simulink model "Motion_planner_Street_Drone"  (R2019b)
settings: Solver=FixedStepAuto  StartTime=0.0  StopTime=25  FixedStep=0.0075  MaxStep=1e-1  MinStep=1e-3  RelTol=1e-3  AbsTol=1e-4
InitFcn:
  | SD_init1
values from neighbouring files (symbols this model uses):
  cost = [2.71432892747 3.32441927977 3.79268757264 4.85642115368 6.12135035287 7.09825974303 9.57278659789 1.55754789407 1.51399555616 2.57723707661 3.8468529147 4.8336387623 ... (2430 elements, 1x2430)]    [matlab.mat]
  Front_brake = [0 2.2085352751 4.15209150797 6.12733711785 8.16604105928 9.79119154879 12.1808659635 14.1242630413 16.1155522836 18.1386900579 20.0839213981 22.1313006548 ... (68 elements, 34x2)]    [Front_brake.mat]
  N = size(X,1)    [curvature.m]
  obsx = [dx1 dx2 dx3 dx4]'    [dynamic_collison.m]    (also in dynamic_detection1.m = [x1 x2 x3 x4]')
  obsy = [dy1 dy2 dy3 dy4]'    [dynamic_collison.m]    (also in dynamic_detection1.m = [y1 y2 y3 y4]')
  x = obs_path(i,1)    [dynamic_collison.m]    (also in dynamic_detection1.m)
  X = [X]    [curvature.m]
  y = obs_path(i,2)    [dynamic_collison.m]    (also in dynamic_detection1.m)
undefined symbols (not defined in the file or in its folder): d, dfin, dini, Ki, Kp, L_0f, lookahead_time, lookahead_time_rev, Rear_brake, sigbuilder_block, steer_ratio, steer_sens, tfin, tini, TPS_0, xfin, Y, yfin, Z
libraries: sm_lib x290, nesl_utility x136, simulink x6, vrlib x2, powerlib_meascontrol x2
(part 1 of 14)
settings Model: PacingRate=0.320000  Creator=dpawa  LastModifiedBy=prave
settings SolverCC: AutoScaleAbsTol=off  InitialStep=1e-2  ZeroCrossAlgorithm=Adaptive  AlgebraicLoopSolver=LineSearch
settings DebuggingCC: AlgebraicLoopMsg=none  MaskedZcDiagnostic=none  IgnoredZcDiagnostic=none  UnderSpecifiedDimensionMsg=warning

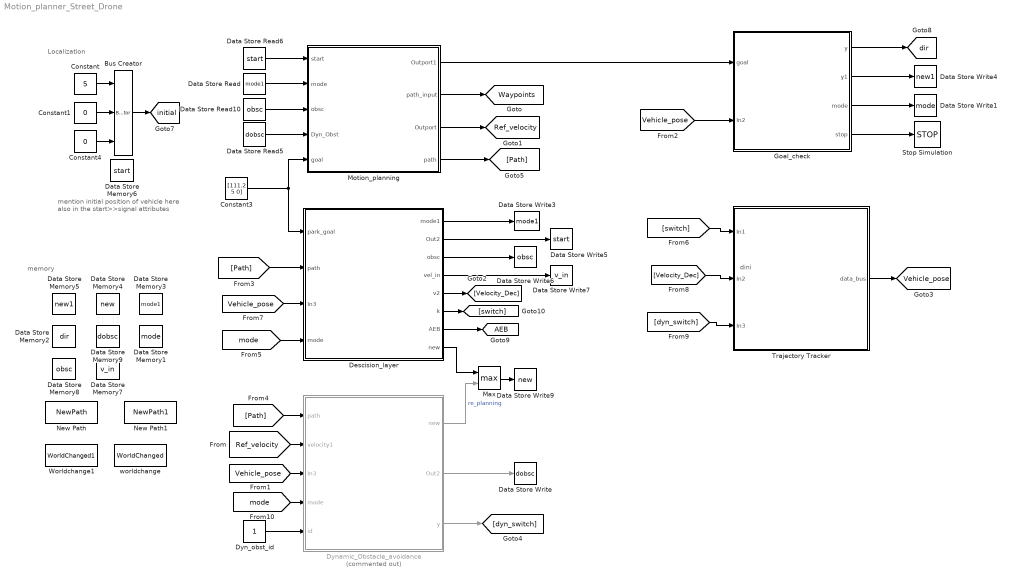
== system Motion_planner_Street_Drone ==
  note: dini
  note: mention initial position of vehicle here
      |  also in the start>>signal attributes
  note: Localization
  note: memory
  Bus Creator : BusCreator  Inputs=3
  Constant : Constant  Value=5
  Constant1 : Constant  Value=0
  Constant3 : Constant  Value=[111.2 5 0]
  Constant4 : Constant  Value=0
  Data Store Memory1 : DataStoreMemory  DataStoreName=mode  ReadBeforeWriteMsg=warning  WriteAfterWriteMsg=warning  WriteAfterReadMsg=warning  InitialValue=1  ShowAdditionalParam=off
  Data Store Memory2 : DataStoreMemory  DataStoreName=dir  ReadBeforeWriteMsg=warning  WriteAfterWriteMsg=warning  WriteAfterReadMsg=warning  InitialValue=1  ShowAdditionalParam=off
  Data Store Memory3 : DataStoreMemory  DataStoreName=mode1  ReadBeforeWriteMsg=warning  WriteAfterWriteMsg=warning  WriteAfterReadMsg=warning  InitialValue=2  ShowAdditionalParam=off  OutDataTypeStr=double
  Data Store Memory4 : DataStoreMemory  DataStoreName=new  ReadBeforeWriteMsg=warning  WriteAfterWriteMsg=warning  WriteAfterReadMsg=warning  ShowAdditionalParam=off  OutDataTypeStr=double
  Data Store Memory5 : DataStoreMemory  DataStoreName=new1  ReadBeforeWriteMsg=warning  WriteAfterWriteMsg=warning  WriteAfterReadMsg=warning  ShowAdditionalParam=off
  Data Store Memory6 : DataStoreMemory  DataStoreName=start  ReadBeforeWriteMsg=warning  WriteAfterWriteMsg=warning  WriteAfterReadMsg=warning  InitialValue=[5 0 0]  ShowAdditionalParam=off  OutDataTypeStr=double
  Data Store Memory7 : DataStoreMemory  DataStoreName=v_in  ReadBeforeWriteMsg=warning  WriteAfterWriteMsg=warning  WriteAfterReadMsg=warning  ShowAdditionalParam=off
  Data Store Memory8 : DataStoreMemory  DataStoreName=obsc  ReadBeforeWriteMsg=warning  WriteAfterWriteMsg=warning  WriteAfterReadMsg=warning  InitialValue=2  ShowAdditionalParam=off
  Data Store Memory9 : DataStoreMemory  DataStoreName=dobsc  ReadBeforeWriteMsg=warning  WriteAfterWriteMsg=warning  WriteAfterReadMsg=warning  InitialValue=[inf inf inf]  ShowAdditionalParam=off
  Data Store Read : DataStoreRead  DataStoreName=mode1
  Data Store Read10 : DataStoreRead  DataStoreName=obsc
  Data Store Read5 : DataStoreRead  DataStoreName=dobsc
  Data Store Read6 : DataStoreRead  DataStoreName=start  SampleTime=0.0075
  Data Store Write : DataStoreWrite  DataStoreName=dobsc
  Data Store Write1 : DataStoreWrite  DataStoreName=mode
  Data Store Write3 : DataStoreWrite  DataStoreName=mode1
  Data Store Write4 : DataStoreWrite  DataStoreName=new1
  Data Store Write5 : DataStoreWrite  DataStoreName=start  SampleTime=0.0075
  Data Store Write6 : DataStoreWrite  DataStoreName=obsc
  Data Store Write7 : DataStoreWrite  DataStoreName=v_in
  Data Store Write9 : DataStoreWrite  DataStoreName=new
  Descision_layer : Subsystem
  Dyn_obst_id : Constant
  Dynamic_Obstacle_avoidance : Subsystem  Commented=on
  Goal_check : Subsystem
  Max : MinMax  Function=max  Inputs=2
  Motion_planning : Subsystem
  "New Path " : DataStoreMemory  DataStoreName=NewPath  ReadBeforeWriteMsg=warning  WriteAfterWriteMsg=warning  WriteAfterReadMsg=warning  VectorParams1D=off  ShowAdditionalParam=off
  New Path1 : DataStoreMemory  DataStoreName=NewPath1  ReadBeforeWriteMsg=warning  WriteAfterWriteMsg=warning  WriteAfterReadMsg=warning  VectorParams1D=off  ShowAdditionalParam=off
  Stop Simulation : Stop
  Trajectory Tracker : Subsystem
  Worldchange1 : DataStoreMemory  DataStoreName=WorldChanged1  VectorParams1D=off  ShowAdditionalParam=off
  worldchange : DataStoreMemory  DataStoreName=WorldChanged  InitialValue=1  VectorParams1D=off  ShowAdditionalParam=off
  tag scope: AEB=global, Ref_velocity=global, Vehicle_pose=global, Waypoints=global, dir=global, initial=global
  wires:
  Constant3/1 -> Descision_layer/1(park_goal), Motion_planning/5(goal)
  Motion_planning/2(path_input) -> [Waypoints]
  Max/1 -> Data Store Write9/1
  [Vehicle_pose] -> Goal_check/2(In2)
  Goal_check/1(y) -> [dir]
  Goal_check/2(y1) -> Data Store Write4/1
  Goal_check/3(mode) -> Data Store Write1/1
  Goal_check/4(stop) -> Stop Simulation/1
  Data Store Read6/1 -> Motion_planning/1(start)
  Data Store Read/1 -> Motion_planning/2(mode)
  Data Store Read10/1 -> Motion_planning/3(obsc)
  Data Store Read5/1 -> Motion_planning/4(Dyn_Obst)
  Motion_planning/3(Outport) -> [Ref_velocity]
  Motion_planning/1(Outport1) -> Goal_check/1(goal)
  Dynamic_Obstacle_avoidance/1(new) -> Max/2  "re_planning"
  [Path] -> Dynamic_Obstacle_avoidance/1(path)
  [Ref_velocity] -> Dynamic_Obstacle_avoidance/2(velocity1)
  [Vehicle_pose] -> Dynamic_Obstacle_avoidance/3(In3)
  [mode] -> Dynamic_Obstacle_avoidance/4(mode)
  Dyn_obst_id/1 -> Dynamic_Obstacle_avoidance/5(id)
  Dynamic_Obstacle_avoidance/2(Out2) -> Data Store Write/1
  [Vehicle_pose] -> Descision_layer/3(In3)
  [mode] -> Descision_layer/4(mode)
  Descision_layer/1(mode1) -> Data Store Write3/1
  Descision_layer/2(Out2) -> Data Store Write5/1
  Descision_layer/3(obsc) -> Data Store Write6/1
  Descision_layer/4(vel_in) -> Data Store Write7/1
  Descision_layer/8(new) -> Max/1
  Constant1/1 -> Bus Creator/2
  Constant/1 -> Bus Creator/1
  Bus Creator/1 -> [initial]
  Constant4/1 -> Bus Creator/3
  Motion_planning/4(path) -> [Path]
  [Path] -> Descision_layer/2(path)
  Descision_layer/5(v2) -> [Velocity_Dec]
  Descision_layer/6(k) -> [switch]
  Dynamic_Obstacle_avoidance/3(y) -> [dyn_switch]
  Descision_layer/7(AEB) -> [AEB]
  [switch] -> Trajectory Tracker/1(In1)
  [Velocity_Dec] -> Trajectory Tracker/2(In2)
  [dyn_switch] -> Trajectory Tracker/3(In3)
  Trajectory Tracker/1(data_bus) -> [Vehicle_pose]

== system Motion_planner_Street_Drone/Descision_layer ==
  park_goal : Inport
  path : Inport  Port=2
  In3 : Inport  Port=3
  mode : Inport  Port=4
  Bus Selector1 : BusSelector  OutputSignals=pos.drive_x,pos.drive_y,angle.yawangle,vel.velocity_drive
  Mux : Mux  Inputs=3
  Subsystem : Subsystem
  mode1 : Outport
  Out2 : Outport  Port=2
  obsc : Outport  Port=3
  vel_in : Outport  Port=4
  v2 : Outport  Port=5
  k : Outport  Port=6
  AEB : Outport  Port=7
  new : Outport  Port=8
  wires:
  Subsystem/5(t_i) -> Mux/3
  Bus Selector1/1 -> Subsystem/3(<drive_x>)  "<drive_x>"
  Subsystem/3(x_i) -> Mux/1
  park_goal/1 -> Subsystem/2(park_goal)
  Subsystem/7(vel_in) -> vel_in/1
  Bus Selector1/3 -> Subsystem/5(<yawangle>)  "<yawangle>"
  Subsystem/4(y_i) -> Mux/2
  In3/1 -> Bus Selector1/1
  Bus Selector1/4 -> Subsystem/6(<velocity_driv e>)  "<velocity_drive>"
  Bus Selector1/2 -> Subsystem/4(<drive_y>)  "<drive_y>"
  Subsystem/2(new) -> new/1
  Subsystem/6(obsc) -> obsc/1
  mode/1 -> Subsystem/7(mode)
  Mux/1 -> Out2/1
  Subsystem/1(y1) -> mode1/1
  Subsystem/8(v2) -> v2/1
  path/1 -> Subsystem/1(path)
  Subsystem/9(k) -> k/1
  Subsystem/10(AEB) -> AEB/1

== system Motion_planner_Street_Drone/Dynamic_Obstacle_avoidance ==
  path : Inport
  velocity1 : Inport  Port=2
  In3 : Inport  Port=3
  mode : Inport  Port=4
  id : Inport  Port=5
  Bus Selector2 : BusSelector  OutputSignals=pos.drive_x,pos.drive_y,angle.yawangle
  MATLAB Function2 : MATLAB Function  TreatAsAtomicUnit=on
  Memory1 : Memory
  Mux1 : Mux  Inputs=2
  Mux2 : Mux  Inputs=3
  Subsystem2 : Subsystem
  Terminator : Terminator
  new : Outport
  Out2 : Outport  Port=2
  y : Outport  Port=3
  wires:
  MATLAB Function2/3(dynobst_y) -> Mux2/2
  Mux1/1 -> Subsystem2/2(In2)
  MATLAB Function2/5(Vel_Dyn) -> Terminator/1
  MATLAB Function2/4(thetad) -> Mux2/3
  Mux2/1 -> Out2/1
  MATLAB Function2/8(y_stop) -> Mux1/2
  Bus Selector2/2 -> MATLAB Function2/4(ya)  "<drive_y>"
  MATLAB Function2/6(dyn_switch) -> Subsystem2/1(u)
  MATLAB Function2/2(dynobst_x) -> Mux2/1
  Memory1/1 -> MATLAB Function2/8("id1 ")
  MATLAB Function2/9(id1) -> Memory1/1
  path/1 -> MATLAB Function2/1(path)
  MATLAB Function2/1(new) -> new/1
  MATLAB Function2/7(x_stop) -> Mux1/1
  Bus Selector2/3 -> MATLAB Function2/5(ta)  "<yawangle>"
  Subsystem2/1(y) -> y/1
  velocity1/1 -> MATLAB Function2/2(velocity1)
  Bus Selector2/1 -> MATLAB Function2/3(xa)  "<drive_x>"
  mode/1 -> MATLAB Function2/6(mode)
  id/1 -> MATLAB Function2/7(id)
  In3/1 -> Bus Selector2/1

== system Motion_planner_Street_Drone/Goal_check ==
  goal : Inport
  In2 : Inport  Port=2
  Bus Selector : BusSelector  OutputSignals=pos.drive_x,pos.drive_y
  Chart1 : Stateflow chart  TreatAsAtomicUnit=on
  MATLAB Function : MATLAB Function  TreatAsAtomicUnit=on
  y : Outport
  y1 : Outport  Port=2
  mode : Outport  Port=3
  stop : Outport  Port=4
  wires:
  Bus Selector/1 -> MATLAB Function/2(x)  "<drive_x>"
  MATLAB Function/1(stop) -> Chart1/1(goal)
  Chart1/4(stop) -> stop/1
  Bus Selector/2 -> MATLAB Function/3(y)  "<drive_y>"
  In2/1 -> Bus Selector/1
  Chart1/1(y) -> y/1
  Chart1/3(mode) -> mode/1
  Chart1/2(y1) -> y1/1
  goal/1 -> MATLAB Function/1(goal)

== system Motion_planner_Street_Drone/Motion_planning ==
  start : Inport
  mode : Inport  Port=2
  obsc : Inport  Port=3
  Dyn_Obst : Inport  Port=4
  goal : Inport  Port=5
  Data Store Read1 : DataStoreRead  DataStoreName=WorldChanged1
  Data Store Read2 : DataStoreRead  DataStoreName=WorldChanged
  Data Store Read3 : DataStoreRead  DataStoreName=mode
  Data Store Read4 : DataStoreRead  DataStoreName=new1
  Data Store Read7 : DataStoreRead  DataStoreName=v_in
  Data Store Read9 : DataStoreRead  DataStoreName=new  DataStoreElements=new
  Motion_Planner : Subsystem  TreatAsAtomicUnit=on
  Pulse Generator : DiscretePulseGenerator  PulseType=Time based  Period=0.015  PulseWidth=50
  Terminator : Terminator
  Transpose : Math  Operator=transpose  SignedPower=off  SaturateOnIntegerOverflow=on
  Velocity_profile : Subsystem
  XOR : Logic  Operator=XOR  IconShape=distinctive  AllPortsSameDT=off  OutDataTypeStr=boolean
  XOR1 : Logic  Operator=XOR  IconShape=distinctive  AllPortsSameDT=off  OutDataTypeStr=boolean
  Outport1 : Outport
  path_input : Outport  Port=2
  Outport : Outport  Port=3
  path : Outport  Port=4
  tag scope: mode=global
  wires:
  Motion_Planner/1(path) -> Velocity_profile/1(path), path/1
  Data Store Read4/1 -> XOR1/1
  Pulse Generator/1 -> Motion_Planner/Trigger
  Data Store Read1/1 -> XOR1/2
  Data Store Read2/1 -> XOR/2
  Data Store Read9/1 -> XOR/1
  Velocity_profile/4(Outport2) -> Terminator/1
  XOR1/1 -> Velocity_profile/Enable
  Data Store Read7/1 -> Velocity_profile/2(In2)
  Velocity_profile/1(path_input) -> Transpose/1
  Data Store Read3/1 -> Velocity_profile/3(mode)
  Motion_Planner/2(Outport) -> [mode]
  Velocity_profile/2(Outport) -> Outport/1
  Dyn_Obst/1 -> Motion_Planner/5(Dyn_Obst)
  start/1 -> Motion_Planner/2(start)
  mode/1 -> Motion_Planner/3(mode)
  goal/1 -> Motion_Planner/1(goal)
  Velocity_profile/3(Outport1) -> Outport1/1
  obsc/1 -> Motion_Planner/4(obsc)
  Transpose/1 -> path_input/1
  XOR/1 -> Motion_Planner/Enable

== system Motion_planner_Street_Drone/Trajectory Tracker ==
  In1 : Inport
  In2 : Inport  Port=2
  In3 : Inport  Port=3
  " Lateral Controller" : Subsystem
  Constant2 : Constant  Value=0
  Constant6 : Constant  Value=0
  Delay : Delay
  First-Order Filter : powerlib_meascontrol/Filters/First-Order Filter  FilterType=Lowpass  Tc=10e-2  Ts=0  Initialize=off  Vac_Init=[0, 0, 60]  Vdc_Init=0  PlotResponse=off  FreqRange="[0,  200,  1]"
  First-Order Filter2 : powerlib_meascontrol/Filters/First-Order Filter  FilterType=Lowpass  Tc=10e-4  Ts=0.0075  Initialize=off  Vac_Init=[0, 0, 60]  Vdc_Init=0  PlotResponse=off  FreqRange="[0,  200,  1]"
  KM- StreetDrone : Subsystem
  Longitudinal Controller : Subsystem
  Scope12 : Scope
  Switch : Switch  Criteria=u2 > Threshold
  Switch1 : Switch  Criteria=u2 > Threshold
  Switch2 : Switch
  input : Subsystem
  save_data_KM : Subsystem
  data_bus : Outport
  wires:
  Switch1/1 -> KM- StreetDrone/1(v_0)
  Longitudinal Controller/1(Velocity) -> First-Order Filter/1
  Delay/1 -> [delta]
  Constant6/1 -> Switch2/3
  [AEB] -> Switch1/2
  Constant2/1 -> Switch1/3
  KM- StreetDrone/1(data_bus) -> data_bus/1, save_data_KM/1(output_bus)
  input/1(Out1) -> [input_bus]
  [Vehicle_pose] -> input/1(data_bus_KM)
  " Lateral Controller"/2(Outport2) -> Switch/1
  First-Order Filter/1 -> Switch1/1
  Switch/1 -> Switch2/1
  First-Order Filter2/1 -> Delay/1
  [Vehicle_pose] -> " Lateral Controller"/2(In2)
  " Lateral Controller"/1(Outport1) -> First-Order Filter2/1
  In3/1 -> Scope12/1, Switch2/2
  [Vehicle_pose] -> Longitudinal Controller/2(In2)
  [input_bus] -> " Lateral Controller"/1(In1)
  Switch2/1 -> Longitudinal Controller/1(ref_velocity)
  In2/1 -> Switch/3
  In1/1 -> Switch/2
  [delta] -> KM- StreetDrone/2(delta)

== system Motion_planner_Street_Drone/Descision_layer/Subsystem ==
  path : Inport
  park_goal : Inport  Port=2
  <drive_x> : Inport  Port=3
  <drive_y> : Inport  Port=4
  <yawangle> : Inport  Port=5
  <velocity_driv e> : Inport  Port=6
  mode : Inport  Port=7
  MATLAB Function2 : MATLAB Function  TreatAsAtomicUnit=on
  y1 : Outport
  new : Outport  Port=2
  x_i : Outport  Port=3
  y_i : Outport  Port=4
  t_i : Outport  Port=5
  obsc : Outport  Port=6
  vel_in : Outport  Port=7
  v2 : Outport  Port=8
  k : Outport  Port=9
  AEB : Outport  Port=10
  wires:
  MATLAB Function2/5(t_i) -> t_i/1
  <drive_x>/1 -> MATLAB Function2/1(xa)
  MATLAB Function2/7(vel_in) -> vel_in/1
  MATLAB Function2/1(mode1) -> y1/1
  mode/1 -> MATLAB Function2/6(mode)
  <yawangle>/1 -> MATLAB Function2/3(ta)
  path/1 -> MATLAB Function2/7(path)
  MATLAB Function2/3(x_i) -> x_i/1
  MATLAB Function2/2(new) -> new/1
  <velocity_driv e>/1 -> MATLAB Function2/5(Vin)
  MATLAB Function2/6(obsc) -> obsc/1
  MATLAB Function2/4(y_i) -> y_i/1
  park_goal/1 -> MATLAB Function2/4(park_goal)
  <drive_y>/1 -> MATLAB Function2/2(ya)
  MATLAB Function2/9(switch1) -> k/1
  MATLAB Function2/8(v2) -> v2/1
  MATLAB Function2/10(AEB) -> AEB/1

== system Motion_planner_Street_Drone/Dynamic_Obstacle_avoidance/Subsystem2 ==
  u : Inport
  In2 : Inport  Port=2
  Bus Selector3 : BusSelector  OutputSignals=pos.drive_x,pos.drive_y
  Chart1 : Stateflow chart  TreatAsAtomicUnit=on
  Delay1 : Delay  DelayLength=1
  Demux : Demux  Outputs=2
  HOLD : MATLAB Function  TreatAsAtomicUnit=on
  Memory2 : Memory  InitialCondition=1
  Stop & GO : MATLAB Function  TreatAsAtomicUnit=on
  Switch1 : Switch
  y : Outport
  wires:
  In2/1 -> Switch1/1
  HOLD/1(y) -> Delay1/1
  Bus Selector3/2 -> Stop & GO/4(y)  "<drive_y>"
  Demux/2 -> Stop & GO/2(stopy)
  Delay1/1 -> Switch1/2
  Switch1/1 -> Demux/1, Memory2/1
  Bus Selector3/1 -> Stop & GO/3(x)  "<drive_x>"
  Demux/1 -> Stop & GO/1(stopx)
  [Vehicle_pose] -> Bus Selector3/1
  Stop & GO/1(stop) -> Chart1/1(stop)
  Memory2/1 -> Switch1/3
  Chart1/1(y) -> y/1
  u/1 -> HOLD/1(u)

== system Motion_planner_Street_Drone/Motion_planning/Motion_Planner ==
  goal : Inport
  start : Inport  Port=2
  mode : Inport  Port=3
  obsc : Inport  Port=4
  Dyn_Obst : Inport  Port=5
  Enable : EnablePort
  Trigger : TriggerPort  VariantControl=Variant  PortDimensions=1
  Constant : Constant  Value=0
  Constant1 : Constant
  Constant10 : Constant  Value=xfin
  Constant11 : Constant  Value=yfin
  Constant12 : Constant  Value=y
  Constant13 : Constant  Value=obsy
  Constant14 : Constant  Value=obsx
  Constant2 : Constant  Value=cost
  Constant3 : Constant  Value=d
  Constant4 : Constant  Value=dfin
  Constant5 : Constant  Value=dini
  Constant6 : Constant  Value=t
  Constant7 : Constant  Value=tfin
  Constant8 : Constant  Value=tini
  Constant9 : Constant  Value=x
  Data Store Write1 : DataStoreWrite  DataStoreName=WorldChanged1
  Data Store Write4 : DataStoreWrite  DataStoreName=WorldChanged
  Gain : Gain  Gain=[1 1 1]
  MATLAB Function : MATLAB Function  TreatAsAtomicUnit=on
  To Workspace : ToWorkspace  VariableName=path  SampleTime=-1
      settings: Save2DSignal=2-D array (concatenate along first dimension)
  To Workspace1 : ToWorkspace  VariableName=path1  SampleTime=-1
      settings: Save2DSignal=2-D array (concatenate along first dimension)
  To Workspace2 : ToWorkspace  VariableName=computational_time  SampleTime=-1
      settings: Save2DSignal=2-D array (concatenate along first dimension)
  path : Outport
  Outport : Outport  Port=2
  wires:
  Constant9/1 -> MATLAB Function/13(x)
  obsc/1 -> MATLAB Function/3(obsc)
  Constant13/1 -> MATLAB Function/5(obsy)
  Constant14/1 -> MATLAB Function/4(obsx)
  Constant6/1 -> MATLAB Function/10(t)
  Constant7/1 -> MATLAB Function/11(tfin)
  Constant8/1 -> MATLAB Function/12(tini)
  Constant11/1 -> MATLAB Function/16(yfin)
  MATLAB Function/1(toctime) -> To Workspace2/1
  Constant2/1 -> MATLAB Function/6(cost)
  Constant4/1 -> MATLAB Function/8(dfin)
  goal/1 -> MATLAB Function/2(goal)
  Constant5/1 -> MATLAB Function/9(dini)
  Constant3/1 -> MATLAB Function/7(d)
  Constant10/1 -> MATLAB Function/14(xfin)
  Constant12/1 -> MATLAB Function/15(y)
  start/1 -> MATLAB Function/1(start)
  MATLAB Function/2(path) -> path/1, To Workspace/1
  mode/1 -> MATLAB Function/17(mode)
  MATLAB Function/3(stop) -> Outport/1
  Constant/1 -> Data Store Write4/1
  Constant1/1 -> Data Store Write1/1
  MATLAB Function/4(steer) -> To Workspace1/1
  Dyn_Obst/1 -> Gain/1
  Gain/1 -> MATLAB Function/18(d_dobst)

== system Motion_planner_Street_Drone/Motion_planning/Velocity_profile ==
  path : Inport
  In2 : Inport  Port=2
  mode : Inport  Port=3
  Enable : EnablePort
  Constant : Constant  Value=0
  Constant1 : Constant
  Constant2 : Constant
  Data Store Write1 : DataStoreWrite  DataStoreName=WorldChanged1
  New Path Available : DataStoreWrite  DataStoreName=NewPath
  New Path Available1 : DataStoreWrite  DataStoreName=NewPath1
  Terminator : Terminator
  To Workspace : ToWorkspace  VariableName=waypoints  SampleTime=-1
      settings: Save2DSignal=2-D array (concatenate along first dimension)
  To Workspace1 : ToWorkspace  VariableName=ref_vel  SampleTime=-1
      settings: Save2DSignal=2-D array (concatenate along first dimension)
  To Workspace2 : ToWorkspace  VariableName=velocity  SampleTime=-1
      settings: Save2DSignal=2-D array (concatenate along first dimension)
  Waypoints : MATLAB Function  TreatAsAtomicUnit=on
  path_input : Outport
  Outport : Outport  Port=2
  Outport1 : Outport  Port=3
  Outport2 : Outport  Port=4
  wires:
  path/1 -> Waypoints/1(path1)
  Waypoints/1(path_input) -> To Workspace/1, path_input/1
  Waypoints/2(velocity) -> To Workspace1/1, Outport/1
  Waypoints/3(goal) -> Outport1/1
  Constant/1 -> Data Store Write1/1
  Waypoints/4(vel1) -> To Workspace2/1, Outport2/1
  Constant1/1 -> New Path Available/1
  Constant2/1 -> New Path Available1/1
  In2/1 -> Waypoints/3(V_in)
  mode/1 -> Waypoints/2(mode)
  Waypoints/5(path_tf) -> Terminator/1

== system Motion_planner_Street_Drone/Trajectory Tracker/ Lateral Controller ==
  In1 : Inport
  In2 : Inport  Port=2
  Bus Selector2 : BusSelector  OutputSignals=positions  OutputAsBus=on
  Bus Selector3 : BusSelector  OutputSignals=vel.velocity_drive  OutputAsBus=on
  Constant1 : Constant  Value=0
  Constant2 : Constant  Value=0
  Fwd_Controller : Subsystem
  Multiport Switch : MultiPortSwitch  DataPortOrder=Specify indices  DataPortIndices={1,0,-1}
  Multiport Switch1 : MultiPortSwitch  DataPortOrder=Specify indices  DataPortIndices={1,0,-1}
  Rev_Controller1 : Subsystem
  Scope{,1..9} (10 alike) : Scope
  Terminator : Terminator
  Terminator1 : Terminator
  Outport1 : Outport
  Outport2 : Outport  Port=2
  wires:
  In2/1 -> Scope6/1, Bus Selector3/1
  Bus Selector2/1 -> Scope1/1, Fwd_Controller/2(positions), Rev_Controller1/1(positions)
  Fwd_Controller/2(distance) -> Terminator1/1
  Bus Selector3/1 -> Scope5/1, Fwd_Controller/1(v_0), Rev_Controller1/2(v_0)
  Rev_Controller1/2(Output) -> Terminator/1
  In1/1 -> Scope/1, Bus Selector2/1
  Fwd_Controller/1(steer angle) -> Scope3/1, Multiport Switch/2
  Multiport Switch/1 -> Outport1/1
  Rev_Controller1/3(steering angle) -> Scope4/1, Multiport Switch/4
  [dir] -> Multiport Switch1/1, Scope2/1, Multiport Switch/1
  Constant1/1 -> Multiport Switch1/3
  Rev_Controller1/1(Velocity) -> Scope9/1, Multiport Switch1/4
  Fwd_Controller/3(Velocity) -> Scope7/1, Multiport Switch1/2
  Multiport Switch1/1 -> Scope8/1, Outport2/1
  Constant2/1 -> Multiport Switch/3

== system Motion_planner_Street_Drone/Trajectory Tracker/KM- StreetDrone ==
  v_0 : Inport
  delta : Inport  Port=2
  Output : Subsystem
  Street_Drone : Subsystem
  data_bus : Outport  VectorParamsAs1DForOutWhenUnconnected=off
  wires:
  delta/1 -> Street_Drone/2(Delta)
  v_0/1 -> Street_Drone/1(Vel)
  Output/1(data_bus) -> data_bus/1

== system Motion_planner_Street_Drone/Trajectory Tracker/Longitudinal Controller ==
  ref_velocity : Inport
  In2 : Inport  Port=2
  Acceleration to Velocity : Subsystem  TreatAsAtomicUnit=on
  Acceleration/ deceleration : Subsystem
  Bus Selector3 : BusSelector  OutputSignals=rate.vel_drive_x,rate.vel_drive_y,angle.yawangle
  MATLAB Function : MATLAB Function  TreatAsAtomicUnit=on
  PID Controller1 : simulink/Continuous/PID Controller  Commented=on  Controller=PI  Form=Ideal  TimeDomain=Continuous-time  SampleTime=0.01  IntegratorMethod=Forward Euler  FilterMethod=Forward Euler  ControllerParametersSource=internal  P=Kp  I=Ki  D=1  UseFilter=on  N=100  TunerSelectOption=Transfer Function Based (PID Tuner App)  ZeroCross=off  InitialConditionSource=internal  InitialConditionForIntegrator=0  InitialConditionForFilter=0  DifferentiatorICPrevScaledInput=0  ExternalReset=none  TrackingMode=off  Kt=1  LimitOutput=on  UpperSaturationLimit=1  LowerSaturationLimit=-2  LinearizeAsGain=off  AntiWindupMode=clamping  Kb=1  POutMin=[]  POutMax=[]  IOutMin=[]  IOutMax=[]  DOutMin=[]  DOutMax=[]  NOutMin=[]  NOutMax=[]  SumOutMin=[]  SumOutMax=[]  SaturationOutMin=[]  SaturationOutMax=[]  PParamMin=[]  PParamMax=[]  IParamMin=[]  IParamMax=[]  DParamMin=[]  DParamMax=[]  NParamMin=[]  NParamMax=[]  KbParamMin=[]  KbParamMax=[]  KtParamMin=[]  KtParamMax=[]  KbOutMin=[]  KbOutMax=[]  KtOutMin=[]  KtOutMax=[]  IntegratorOutMin=[]  IntegratorOutMax=[]  FilterOutMin=[]  FilterOutMax=[]  SumI1OutMin=[]  SumI1OutMax=[]  SumI2OutMin=[]  SumI2OutMax=[]  SumI3OutMin=[]  SumI3OutMax=[]  SumI4OutMin=[]  SumI4OutMax=[]  SumDOutMin=[]  SumDOutMax=[]  DifferentiatorOutMin=[]  DifferentiatorOutMax=[]  FilterDiffOutCoefMin=[]  FilterDiffOutCoefMax=[]  ReciprocalOutMin=[]  ReciprocalOutMax=[]  SumDenOutMin=[]  SumDenOutMax=[]  SumNumOutMin=[]  SumNumOutMax=[]  DivideOutMin=[]  DivideOutMax=[]  IntegratorContinuousStateAttributes=''  IntegratorStateMustResolveToSignalObject=off  IntegratorRTWStateStorageClass=Auto  FilterContinuousStateAttributes=''  FilterStateMustResolveToSignalObject=off  FilterRTWStateStorageClass=Auto  ParallelPVariant=Passthrough  IdealPVariant=InternalParameters  IVariant=InternalParameters  DVariant=Disabled  IntegratorVariant=Continuous  SatVariant=Enabled  AWVariant=ContClampingIdeal  PCopyVariant=InternalParamsIdeal  TRVariant=Disabled  FdbkBlocksVariant=Forward  IdealPFdbkVariant=Disabled  SatFdbkVariant=Disabled  DerivativeFilterVariant=Disabled  NVariant=Disabled  NCopyVariant=Disabled_SignalSpec  FilterICVariant=Disabled  IntegratorICVariant=InternalICs  ExternalResetVariant=Disabled  TRSumVariant=Passthrough  SumFdbkVariant=Disabled  SumVariant=Sum_PI
  PID Controller2 : simulink/Continuous/PID Controller  Controller=PI  Form=Ideal  TimeDomain=Continuous-time  SampleTime=0.01  IntegratorMethod=Forward Euler  FilterMethod=Forward Euler  ControllerParametersSource=internal  P=Kp  I=Ki  D=1  UseFilter=on  N=100  TunerSelectOption=Transfer Function Based (PID Tuner App)  ZeroCross=off  InitialConditionSource=internal  InitialConditionForIntegrator=0  InitialConditionForFilter=0  DifferentiatorICPrevScaledInput=0  ExternalReset=none  TrackingMode=off  Kt=1  LimitOutput=on  UpperSaturationLimit=2  LowerSaturationLimit=-6  LinearizeAsGain=off  AntiWindupMode=clamping  Kb=1  POutMin=[]  POutMax=[]  IOutMin=[]  IOutMax=[]  DOutMin=[]  DOutMax=[]  NOutMin=[]  NOutMax=[]  SumOutMin=[]  SumOutMax=[]  SaturationOutMin=[]  SaturationOutMax=[]  PParamMin=[]  PParamMax=[]  IParamMin=[]  IParamMax=[]  DParamMin=[]  DParamMax=[]  NParamMin=[]  NParamMax=[]  KbParamMin=[]  KbParamMax=[]  KtParamMin=[]  KtParamMax=[]  KbOutMin=[]  KbOutMax=[]  KtOutMin=[]  KtOutMax=[]  IntegratorOutMin=[]  IntegratorOutMax=[]  FilterOutMin=[]  FilterOutMax=[]  SumI1OutMin=[]  SumI1OutMax=[]  SumI2OutMin=[]  SumI2OutMax=[]  SumI3OutMin=[]  SumI3OutMax=[]  SumI4OutMin=[]  SumI4OutMax=[]  SumDOutMin=[]  SumDOutMax=[]  DifferentiatorOutMin=[]  DifferentiatorOutMax=[]  FilterDiffOutCoefMin=[]  FilterDiffOutCoefMax=[]  ReciprocalOutMin=[]  ReciprocalOutMax=[]  SumDenOutMin=[]  SumDenOutMax=[]  SumNumOutMin=[]  SumNumOutMax=[]  DivideOutMin=[]  DivideOutMax=[]  IntegratorContinuousStateAttributes=''  IntegratorStateMustResolveToSignalObject=off  IntegratorRTWStateStorageClass=Auto  FilterContinuousStateAttributes=''  FilterStateMustResolveToSignalObject=off  FilterRTWStateStorageClass=Auto  ParallelPVariant=Passthrough  IdealPVariant=InternalParameters  IVariant=InternalParameters  DVariant=Disabled  IntegratorVariant=Continuous  SatVariant=Enabled  AWVariant=ContClampingIdeal  PCopyVariant=InternalParamsIdeal  TRVariant=Disabled  FdbkBlocksVariant=Forward  IdealPFdbkVariant=Disabled  SatFdbkVariant=Disabled  DerivativeFilterVariant=Disabled  NVariant=Disabled  NCopyVariant=Disabled_SignalSpec  FilterICVariant=Disabled  IntegratorICVariant=InternalICs  ExternalResetVariant=Disabled  TRSumVariant=Passthrough  SumFdbkVariant=Disabled  SumVariant=Sum_PI
  Scope{1..2,4..6} (5 alike) : Scope
  Scope3 : Scope  NumInputPorts=3
  Subtract : Sum  Inputs=+-
  To Workspace : ToWorkspace  VariableName=actual  SampleTime=-1
      settings: Save2DSignal=2-D array (concatenate along first dimension)
  Velocity : Outport
  wires:
  Acceleration/ deceleration/1(Out1) -> Acceleration to Velocity/2(AccelCmd)
  ref_velocity/1 -> Scope1/1, To Workspace/1, Subtract/1
  Bus Selector3/3 -> Scope3/3, MATLAB Function/3(t)  "<yawangle>"
  Acceleration/ deceleration/2(Out2) -> Acceleration to Velocity/3(DecelCmd)
  Bus Selector3/1 -> Scope3/1, MATLAB Function/1(ux)  "<vel_drive_x>"
  Subtract/1 -> Scope2/1, PID Controller2/1
  [dir] -> Acceleration/ deceleration/1(In1), Acceleration to Velocity/1(Direction)
  Bus Selector3/2 -> Scope3/2, MATLAB Function/2(uy)  "<vel_drive_y>"
  In2/1 -> Scope4/1, Bus Selector3/1
  PID Controller2/1 -> Scope6/1, Acceleration/ deceleration/2(In2)
  MATLAB Function/1(y) -> Scope5/1, Subtract/2
  Acceleration to Velocity/1(Velocity) -> Velocity/1

== system Motion_planner_Street_Drone/Trajectory Tracker/input ==
  data_bus_KM : Inport
  Bus Creator : BusCreator  Inputs=2
  Bus Selector : BusSelector  OutputSignals=pos.drive_x,pos.drive_y
  Bus Selector1 : BusSelector  OutputSignals=pos.x_0f,pos.y_0f
  Constant : Constant
  Constant1 : Constant  Value=0
  Constant3 : Constant  Value=0
  Multiport Switch : MultiPortSwitch  DataPortOrder=Specify indices  DataPortIndices={-1,0,1}
  Mux : Mux  Inputs=3
  Mux1 : Mux  Inputs=3
  Mux2 : Mux  Inputs=2
  Mux3 : Mux  Inputs=2
  Scope{,1..10} (11 alike) : Scope
  Out1 : Outport  VectorParamsAs1DForOutWhenUnconnected=off
  wires:
  Bus Creator/1 -> Scope10/1, Out1/1
  Constant1/1 -> Mux/3
  Constant3/1 -> Mux1/3
  data_bus_KM/1 -> Bus Selector/1, Bus Selector1/1
  Bus Selector/1 -> Scope/1, Mux/1  "<drive_x>"
  Bus Selector/2 -> Mux/2, Scope1/1  "<drive_y>"
  Bus Selector1/1 -> Scope3/1, Mux1/1  "<x_0f>"
  Bus Selector1/2 -> Scope2/1, Mux1/2  "<y_0f>"
  Mux1/1 -> Mux3/2, Mux2/1, Scope5/1  "Steer_axle"
  Multiport Switch/1 -> Scope8/1, Bus Creator/2  "positions"
  Mux/1 -> Scope4/1, Mux3/1, Mux2/2  "drive_axle"
  Constant/1 -> Bus Creator/1
  Mux3/1 -> Scope7/1, Multiport Switch/3, Multiport Switch/2  "position_input_rev_controller"
  [dir] -> Scope9/1, Multiport Switch/1
  Mux2/1 -> Scope6/1, Multiport Switch/4  "position_input_fwd_controller"

== system Motion_planner_Street_Drone/Trajectory Tracker/save_data_KM ==
  output_bus : Inport
  Bus Selector : BusSelector  OutputSignals=pos.drive_x,pos.drive_y,pos.x_0f,pos.y_0f  OutputAsBus=on
  Bus Selector1 : BusSelector  OutputSignals=rate.yawrate,rate.vel_drive_x,rate.vel_drive_y  OutputAsBus=on
  Bus Selector2 : BusSelector  OutputSignals=angle.yawangle,angle.steering_angle  OutputAsBus=on
  Bus Selector3 : BusSelector  OutputSignals=vel.velocity_drive  OutputAsBus=on
  To Workspace14 : ToWorkspace  VariableName=SD_rate  SampleTime=-1
      settings: Save2DSignal=2-D array (concatenate along first dimension)
  To Workspace15 : ToWorkspace  VariableName=SD_angle  SampleTime=-1
      settings: Save2DSignal=2-D array (concatenate along first dimension)
  To Workspace17 : ToWorkspace  VariableName=SD_vel  SampleTime=-1
      settings: Save2DSignal=2-D array (concatenate along first dimension)
  To Workspace9 : ToWorkspace  VariableName=SD_pos  SampleTime=-1
      settings: Save2DSignal=2-D array (concatenate along first dimension)
  wires:
  output_bus/1 -> Bus Selector2/1, Bus Selector3/1, Bus Selector/1, Bus Selector1/1
  Bus Selector1/1 -> To Workspace14/1  "rate"
  Bus Selector/1 -> To Workspace9/1  "pos"
  Bus Selector3/1 -> To Workspace17/1  "vel"
  Bus Selector2/1 -> To Workspace15/1  "angle"

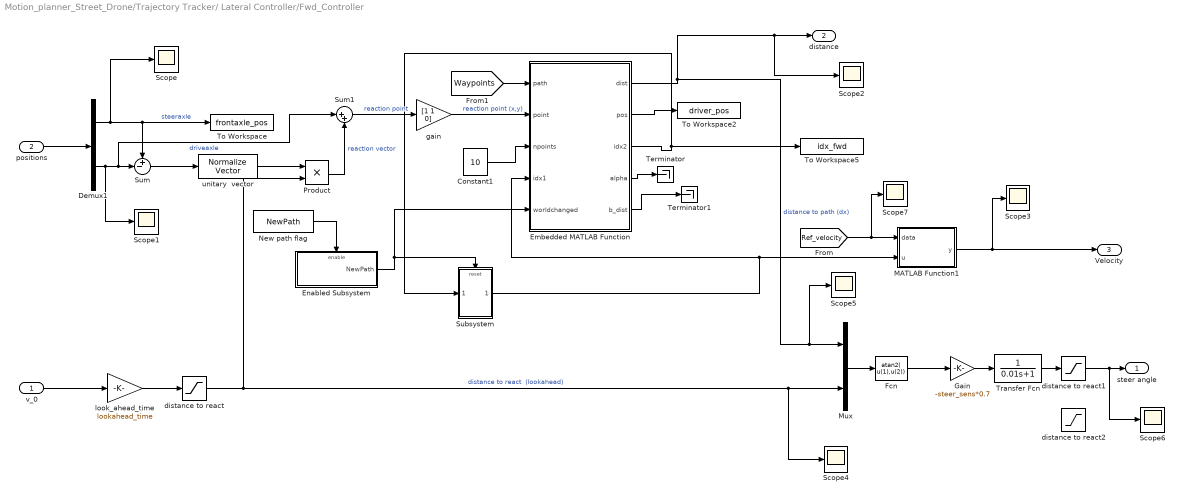
== system Motion_planner_Street_Drone/Trajectory Tracker/ Lateral Controller/Fwd_Controller ==
  v_0 : Inport
  positions : Inport  Port=2
  Constant1 : Constant  Value=10
  Demux1 : Demux  Outputs=2
  Embedded MATLAB Function : MATLAB Function  TreatAsAtomicUnit=on  SystemSampleTime=[0.0075 0]
  Enabled Subsystem : Subsystem  TreatAsAtomicUnit=on
  Fcn : Fcn  Expr=atan2( u(1),u(2))
  Gain : Gain  Gain=-steer_sens*0.7
  MATLAB Function1 : MATLAB Function  TreatAsAtomicUnit=on
  Mux : Mux  Inputs=2
  New path flag : DataStoreRead  DataStoreName=NewPath
  Product : Product  RndMeth=Zero
  Scope{,1..7} (8 alike) : Scope
  Subsystem : Subsystem
  Sum : Sum  Inputs=+-|
  Sum1 : Sum  Inputs=|++
  Terminator : Terminator
  Terminator1 : Terminator
  To Workspace : ToWorkspace  VariableName=frontaxle_pos  SampleTime=-1
  To Workspace2 : ToWorkspace  VariableName=driver_pos  SampleTime=-1
  To Workspace5 : ToWorkspace  VariableName=idx_fwd  SampleTime=-1
  Transfer Fcn : TransferFcn  Denominator=[0.01 1]
  distance to react : Saturate  UpperLimit=100  LowerLimit=0.5
  distance to react1 : Saturate  UpperLimit=0.15  LowerLimit=-0.1
  distance to react2 : Saturate  UpperLimit=0.53  LowerLimit=-0.53
  gain : Gain  Gain=[1 1 0]
  look_ahead_time : Gain  Gain=lookahead_time
  "unitary  vector " : vrlib/Utilities/Normalize Vector  maxzero=0
  steer angle : Outport
  distance : Outport  Port=2
  Velocity : Outport  Port=3
  wires:
  Gain/1 -> Transfer Fcn/1
  Demux1/2 -> Scope1/1, Sum1/1, Sum/2  "driveaxle"
  Sum1/1 -> gain/1  "reaction point"
  v_0/1 -> look_ahead_time/1
  [Waypoints] -> Embedded MATLAB Function/1(path)
  look_ahead_time/1 -> distance to react/1
  Product/1 -> Sum1/2  "reaction vector"
  distance to react/1 -> Scope4/1, Mux/2, Product/2  "distance to react  (lookahead)"
  Embedded MATLAB Function/5(b_dist) -> Terminator1/1
  Sum/1 -> "unitary  vector "/1
  positions/1 -> Demux1/1
  gain/1 -> Embedded MATLAB Function/2(point)  "reaction point (x,y)"
  Embedded MATLAB Function/2(pos) -> To Workspace2/1
  Constant1/1 -> Embedded MATLAB Function/3(npoints)
  Transfer Fcn/1 -> distance to react1/1
  Embedded MATLAB Function/4(alpha) -> Terminator/1
  Demux1/1 -> Scope/1, To Workspace/1, Sum/1  "steeraxle"
  Mux/1 -> Fcn/1
  Embedded MATLAB Function/1(dist) -> Scope2/1, distance/1, Scope5/1, Mux/1  "distance to path (dx)"
  "unitary  vector "/1 -> Product/1
  distance to react1/1 -> Scope6/1, steer angle/1
  Fcn/1 -> Gain/1
  [Ref_velocity] -> Scope7/1, MATLAB Function1/1(data)
  MATLAB Function1/1(y) -> Scope3/1, Velocity/1
  Enabled Subsystem/1(NewPath) -> Embedded MATLAB Function/5(worldchanged), Subsystem/Reset
  New path flag/1 -> Enabled Subsystem/Enable
  Subsystem/1(indice dans le parcours) -> MATLAB Function1/2(u), Embedded MATLAB Function/4(idx1)
  Embedded MATLAB Function/3(idx2) -> To Workspace5/1, Subsystem/1(In1)

== system Motion_planner_Street_Drone/Trajectory Tracker/ Lateral Controller/Rev_Controller1 ==
  positions : Inport
  v_0 : Inport  Port=2
  Constant1 : Constant  Value=10
  Demux1 : Demux  Outputs=2
  Embedded MATLAB Function : MATLAB Function  TreatAsAtomicUnit=on
  Enabled Subsystem : Subsystem  TreatAsAtomicUnit=on
  Fcn : Fcn  Expr=atan2( u(1),u(2))
  Gain : Gain  Gain=steer_sens*steer_ratio
  MATLAB Function1 : MATLAB Function  TreatAsAtomicUnit=on
  Mux : Mux  Inputs=2
  New path flag : DataStoreRead  DataStoreName=NewPath1
  Product : Product  RndMeth=Zero
  Resettable Subsystem : Subsystem  TreatAsAtomicUnit=on
  Sum : Sum  Inputs=+-|
  Sum1 : Sum  Inputs=|++
  Terminator : Terminator
  Terminator1 : Terminator
  To Workspace : ToWorkspace  VariableName=frontaxle_pos_rev  SaveFormat=Structure  SampleTime=-1
  To Workspace1 : ToWorkspace  VariableName=driver_viewpoint_rev  SaveFormat=Structure  SampleTime=-1
  To Workspace2 : ToWorkspace  VariableName=driver_pos_rev  SampleTime=-1
  Transfer Fcn : TransferFcn  Denominator=[0.01 1]
  distance to react : Saturate  UpperLimit=100  LowerLimit=0.5
  distance to react1 : Saturate  UpperLimit=0.53  LowerLimit=-0.53
  gain : Gain  Gain=[1 1 0]
  look_ahead_time : Gain  Gain=lookahead_time_rev
  "unitary truck vector " : vrlib/Utilities/Normalize Vector  maxzero=0
  Velocity : Outport
  Output : Outport  Port=2
  steering angle : Outport  Port=3
  wires:
  distance to react1/1 -> steering angle/1
  look_ahead_time/1 -> distance to react/1
  Embedded MATLAB Function/2(pos) -> To Workspace2/1
  Embedded MATLAB Function/5(b_dist) -> Terminator1/1
  positions/1 -> Demux1/1
  distance to react/1 -> Product/2, Mux/2  "distance to react  (lookahead)"
  Transfer Fcn/1 -> distance to react1/1
  Mux/1 -> Fcn/1
  Constant1/1 -> Embedded MATLAB Function/3(npoints)
  Embedded MATLAB Function/3(idx2) -> Resettable Subsystem/1(In1)
  Embedded MATLAB Function/1(dist) -> Output/1, Mux/1  "distance to path (dx)"
  Embedded MATLAB Function/4(alpha) -> Terminator/1
  Demux1/2 -> Sum/2  "driveaxle"
  "unitary truck vector "/1 -> Product/1
  Fcn/1 -> Gain/1
  Product/1 -> Sum1/2  "reaction vector"
  gain/1 -> To Workspace1/1, Embedded MATLAB Function/2(point)  "reaction point (x,y)"
  v_0/1 -> look_ahead_time/1
  Sum/1 -> "unitary truck vector "/1  "truck vector"
  Sum1/1 -> gain/1  "reaction point"
  Demux1/1 -> Sum/1, Sum1/1, To Workspace/1  "steeraxle"
  Gain/1 -> Transfer Fcn/1
  [Ref_velocity] -> MATLAB Function1/1(data)
  MATLAB Function1/1(y) -> Velocity/1
  [Waypoints] -> Embedded MATLAB Function/1(path)
  Enabled Subsystem/1(NewPath) -> Embedded MATLAB Function/5(worldchanged), Resettable Subsystem/Reset
  New path flag/1 -> Enabled Subsystem/Enable
  Resettable Subsystem/1(idx1) -> MATLAB Function1/2(u), Embedded MATLAB Function/4(idx1)  "indice"

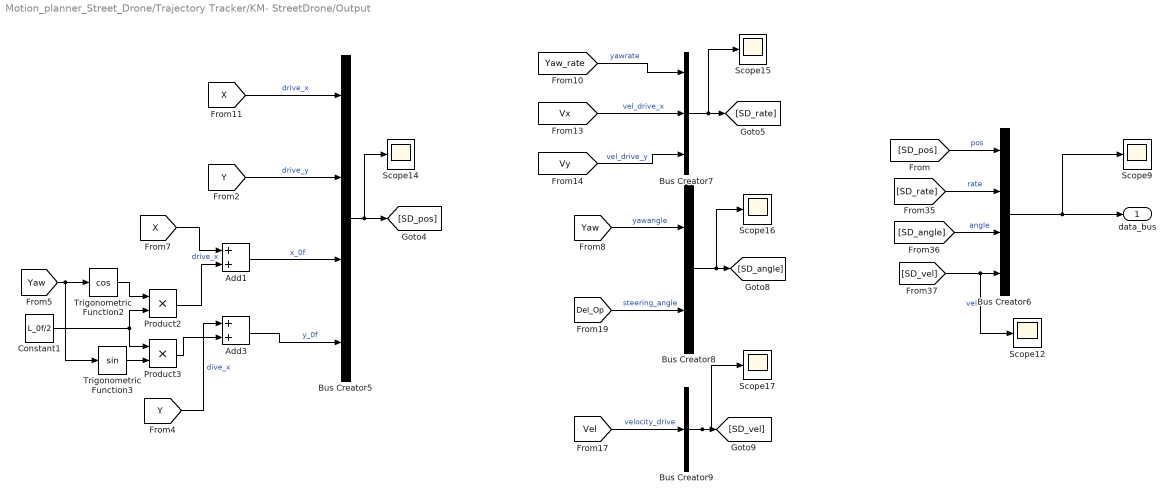
== system Motion_planner_Street_Drone/Trajectory Tracker/KM- StreetDrone/Output ==
  Add1 : Sum
  Add3 : Sum
  Bus Creator5 : BusCreator  Inputs=4
  Bus Creator6 : BusCreator  Inputs=4
  Bus Creator7 : BusCreator  Inputs=3
  Bus Creator8 : BusCreator  Inputs=2
  Bus Creator9 : BusCreator  Inputs=1
  Constant1 : Constant  Value=L_0f/2
  Product2 : Product
  Product3 : Product
  Scope{9,12,14..17} (6 alike) : Scope
  Trigonometric Function2 : Trigonometry  Operator=cos
  Trigonometric Function3 : Trigonometry
  data_bus : Outport  VectorParamsAs1DForOutWhenUnconnected=off
  wires:
  Bus Creator9/1 -> Scope17/1, [SD_vel]
  Product3/1 -> Add3/2
  [Y] -> Bus Creator5/2  "drive_y"
  [SD_angle] -> Bus Creator6/3  "angle"
  Bus Creator7/1 -> [SD_rate], Scope15/1
  [SD_pos] -> Bus Creator6/1  "pos"
  Bus Creator6/1 -> data_bus/1, Scope9/1
  [SD_vel] -> Scope12/1, Bus Creator6/4  "vel"
  [SD_rate] -> Bus Creator6/2  "rate"
  Trigonometric Function2/1 -> Product2/1
  [Del_Op] -> Bus Creator8/2  "steering_angle"
  [Yaw] -> Bus Creator8/1  "yawangle"
  [Yaw] -> Trigonometric Function2/1, Trigonometric Function3/1
  [X] -> Bus Creator5/1  "drive_x"
  [Vy] -> Bus Creator7/3  "vel_drive_y"
  Bus Creator8/1 -> [SD_angle], Scope16/1
  Add1/1 -> Bus Creator5/3  "x_0f"
  [Vx] -> Bus Creator7/2  "vel_drive_x"
  Bus Creator5/1 -> [SD_pos], Scope14/1
  Constant1/1 -> Product2/2, Product3/1
  Trigonometric Function3/1 -> Product3/2
  [Vel] -> Bus Creator9/1  "velocity_drive"
  [Y] -> Add3/1  "dive_x"
  [X] -> Add1/1  "drive_x"
  Add3/1 -> Bus Creator5/4  "y_0f"
  Product2/1 -> Add1/2
  [Yaw_rate] -> Bus Creator7/1  "yawrate"

== system Motion_planner_Street_Drone/Trajectory Tracker/KM- StreetDrone/Street_Drone ==
  Vel : Inport
  Delta : Inport  Port=2
  Gearbox : Subsystem
  Inputs : Subsystem
  Powertrain and Brake System1 : Subsystem
  Results1 : Subsystem
  Vehicle : Subsystem
  wires:
  Vel/1 -> Inputs/2(Vel)
  Delta/1 -> Inputs/1(Delta)

== system Motion_planner_Street_Drone/Trajectory Tracker/Longitudinal Controller/Acceleration to Velocity ==
  Direction : Inport
  AccelCmd : Inport  Port=2  PortDimensions=[1 1]
  DecelCmd : Inport  Port=3  PortDimensions=[1 1]
  AND : Logic  IconShape=distinctive  AllPortsSameDT=off  OutDataTypeStr=boolean
  Abs : Abs
  Add : Sum  Inputs=+-
  Compare To Zero : simulink/Logic and Bit Operations/Compare To Zero  relop=<=  OutDataTypeStr=boolean
  Compare To Zero1 : simulink/Logic and Bit Operations/Compare To Zero  relop=>  OutDataTypeStr=boolean
  Constant : Constant  Value=0.01
  Constant1 : Constant  Value=0
  Minus : Sum  Inputs=+-
  Product1 : Product
  Saturated integrator : Integrator  ExternalReset=either  LimitOutput=on  LowerSaturationLimit=0  AbsoluteTolerance=1e-3  ZeroCross=off
  Saturation : Saturate  UpperLimit=20  LowerLimit=0
  Scope : Scope
  Scope6 : Scope
  Switch : Switch  Criteria=u2 > Threshold
  Unit Delay : UnitDelay  SampleTime=-1  HasFrameUpgradeWarning=on
  Unit Delay1 : UnitDelay  Commented=on  SampleTime=0.01  HasFrameUpgradeWarning=on
  Velocity : Outport  VectorParamsAs1DForOutWhenUnconnected=off
  wires:
  Direction/1 -> Product1/2, Saturated integrator/2
  AccelCmd/1 -> Add/1
  Add/1 -> Scope/1, Saturated integrator/1
  DecelCmd/1 -> Compare To Zero1/1, Add/2
  Unit Delay/1 -> Abs/1
  Abs/1 -> Minus/1
  Constant/1 -> Minus/2
  Minus/1 -> Compare To Zero/1
  Compare To Zero/1 -> AND/2
  Compare To Zero1/1 -> AND/1
  AND/1 -> Switch/2  "Reset velocity to zero"
  Switch/1 -> Unit Delay/1, Saturation/1
  Constant1/1 -> Switch/1
  Saturated integrator/1 -> Product1/1
  Product1/1 -> Switch/3
  Saturation/1 -> Scope6/1, Velocity/1

== system Motion_planner_Street_Drone/Trajectory Tracker/Longitudinal Controller/Acceleration// deceleration ==
  In1 : Inport
  In2 : Inport  Port=2
  Abs : Abs
  Constant1 : Constant  Value=0  VectorParams1D=off  SampleTime=-1
  Multiply : Product
  Reset Specification1 : SignalSpecification  SampleTime=0.0075
  Reset Specification2 : SignalSpecification  Commented=on  SampleTime=0.01
  Scope{1..3,6} (4 alike) : Scope
  Switch : Switch  Criteria=u2 > Threshold
  Switch1 : Switch  Criteria=u2 > Threshold
  Out1 : Outport
  Out2 : Outport  Port=2
  wires:
  Switch/1 -> Scope1/1, Out1/1
  In1/1 -> Multiply/1
  Constant1/1 -> Reset Specification1/1
  Switch1/1 -> Scope2/1, Out2/1
  Reset Specification1/1 -> Switch/3, Switch1/1
  Abs/1 -> Scope3/1, Switch1/3
  Multiply/1 -> Scope6/1, Abs/1, Switch1/2, Switch/1, Switch/2
  In2/1 -> Multiply/2

== system Motion_planner_Street_Drone/Trajectory Tracker/ Lateral Controller/Fwd_Controller/Enabled Subsystem ==
  Enable : EnablePort  ZeroCross=off
  Constant : Constant
  Constant1 : Constant  Value=0
  New path flag : DataStoreWrite  DataStoreName=NewPath
  NewPath : Outport  OutputWhenDisabled=reset  InitialOutput=0  VectorParamsAs1DForOutWhenUnconnected=off
  wires:
  Constant/1 -> NewPath/1
  Constant1/1 -> New path flag/1

== system Motion_planner_Street_Drone/Trajectory Tracker/ Lateral Controller/Fwd_Controller/Subsystem ==
  In1 : Inport
  Reset : ResetPort  DisableCoverage=on
  Memory : Memory  InitialCondition=-1
  indice dans le parcours : Outport
  wires:
  Memory/1 -> indice dans le parcours/1  "indice dans le parcours"
  In1/1 -> Memory/1

== system Motion_planner_Street_Drone/Trajectory Tracker/ Lateral Controller/Rev_Controller1/Enabled Subsystem ==
  Enable : EnablePort  ZeroCross=off
  Constant : Constant
  Constant1 : Constant  Value=0
  New path flag : DataStoreWrite  DataStoreName=NewPath1
  NewPath : Outport  OutputWhenDisabled=reset  InitialOutput=0  VectorParamsAs1DForOutWhenUnconnected=off
  wires:
  Constant/1 -> NewPath/1
  Constant1/1 -> New path flag/1

== system Motion_planner_Street_Drone/Trajectory Tracker/ Lateral Controller/Rev_Controller1/Resettable Subsystem ==
  In1 : Inport
  Reset : ResetPort  DisableCoverage=on
  Memory : Memory  InitialCondition=-1
  idx1 : Outport
  wires:
  In1/1 -> Memory/1
  Memory/1 -> idx1/1  "indice dans le parcours"

== system Motion_planner_Street_Drone/Trajectory Tracker/KM- StreetDrone/Street_Drone/Gearbox ==
  Constant : Constant  Value=0
  For_reverse : Gain  Gain=-1
  Manual Switch1 : ManualSwitch  CurrentSetting=0
  Manual Switch2 : ManualSwitch
  tag scope: tau=global
  wires:
  For_reverse/1 -> Manual Switch2/2
  Manual Switch2/1 -> Manual Switch1/2
  [final_tau] -> Manual Switch2/1, For_reverse/1
  Constant/1 -> Manual Switch1/1
  Manual Switch1/1 -> [tau]

== system Motion_planner_Street_Drone/Trajectory Tracker/KM- StreetDrone/Street_Drone/Inputs ==
  Delta : Inport
  Vel : Inport  Port=2
  Del : Subsystem
  Velocity : Subsystem
  wires:
  Delta/1 -> Del/1(del)
  Vel/1 -> Velocity/1(Vel)

== system Motion_planner_Street_Drone/Trajectory Tracker/KM- StreetDrone/Street_Drone/Powertrain and Brake System1 ==
  Abs : Abs
  Brake_system : Subsystem
  Divide : Product  Inputs=/*
  Driveline_viscous_losses : Subsystem
  Gain1 : Gain  Gain=0.5
  Gear_ratio : Gain  Gain=9.23
  Motor : Subsystem
  PI Controller : simulink/Continuous/PID Controller  Controller=PID  Form=Parallel  TimeDomain=Continuous-time  SampleTime=-1  IntegratorMethod=Forward Euler  FilterMethod=Forward Euler  ControllerParametersSource=internal  P=150  I=1  D=0  UseFilter=on  N=100  TunerSelectOption=Transfer Function Based (PID Tuner App)  InitialConditionSource=internal  InitialConditionForIntegrator=0  InitialConditionForFilter=0  DifferentiatorICPrevScaledInput=0  ExternalReset=none  TrackingMode=off  Kt=1  LimitOutput=off  UpperSaturationLimit=inf  LowerSaturationLimit=-inf  LinearizeAsGain=on  AntiWindupMode=none  Kb=1  POutMin=[]  POutMax=[]  IOutMin=[]  IOutMax=[]  DOutMin=[]  DOutMax=[]  NOutMin=[]  NOutMax=[]  SumOutMin=[]  SumOutMax=[]  SaturationOutMin=[]  SaturationOutMax=[]  PParamMin=[]  PParamMax=[]  IParamMin=[]  IParamMax=[]  DParamMin=[]  DParamMax=[]  NParamMin=[]  NParamMax=[]  KbParamMin=[]  KbParamMax=[]  KtParamMin=[]  KtParamMax=[]  KbOutMin=[]  KbOutMax=[]  KtOutMin=[]  KtOutMax=[]  IntegratorOutMin=[]  IntegratorOutMax=[]  FilterOutMin=[]  FilterOutMax=[]  SumI1OutMin=[]  SumI1OutMax=[]  SumI2OutMin=[]  SumI2OutMax=[]  SumI3OutMin=[]  SumI3OutMax=[]  SumI4OutMin=[]  SumI4OutMax=[]  SumDOutMin=[]  SumDOutMax=[]  DifferentiatorOutMin=[]  DifferentiatorOutMax=[]  FilterDiffOutCoefMin=[]  FilterDiffOutCoefMax=[]  ReciprocalOutMin=[]  ReciprocalOutMax=[]  SumDenOutMin=[]  SumDenOutMax=[]  SumNumOutMin=[]  SumNumOutMax=[]  DivideOutMin=[]  DivideOutMax=[]  IntegratorContinuousStateAttributes=''  IntegratorStateMustResolveToSignalObject=off  IntegratorRTWStateStorageClass=Auto  FilterContinuousStateAttributes=''  FilterStateMustResolveToSignalObject=off  FilterRTWStateStorageClass=Auto  ParallelPVariant=InternalParameters  IdealPVariant=Disabled  IVariant=InternalParameters  DVariant=InternalParameters  IntegratorVariant=Continuous  SatVariant=Disabled  AWVariant=Passthrough  PCopyVariant=Disabled  TRVariant=Disabled  FdbkBlocksVariant=Forward  IdealPFdbkVariant=Disabled  SatFdbkVariant=Disabled  DerivativeFilterVariant=ContFilter  NVariant=InternalParameters  NCopyVariant=Disabled  FilterICVariant=InternalICsFilter  IntegratorICVariant=InternalICs  ExternalResetVariant=Disabled  TRSumVariant=Passthrough  SumFdbkVariant=Disabled  SumVariant=Sum_PID
  Rate Limiter6 : RateLimiter  RisingSlewLimit=600  FallingSlewLimit=-1000  SampleTimeMode=inherited
  Scaling : Subsystem
  Scope{,1,3,19,24} (5 alike) : Scope
  Scope18 : Scope  NumInputPorts=2
  Subtract : Sum  Inputs=+-
  Subtract2 : Sum  Inputs=+-
  To Workspace : ToWorkspace  VariableName=Desired_Vel  SampleTime=-1
  To Workspace1 : ToWorkspace  VariableName=Motor_force  SampleTime=-1
  tag scope: Me_Pt=global, final_tau=global
  wires:
  Rate Limiter6/1 -> [Me_Pt], Divide/2, Scope/1, [final_tau]
  Abs/1 -> Scope18/2, Subtract/2, Motor/1(I/p2)  "Actual"
  Gain1/1 -> Rate Limiter6/1
  Divide/1 -> Scope1/1, To Workspace1/1
  [RL_Re] -> Divide/1
  Scaling/1(O/p) -> Gain1/1
  Gear_ratio/1 -> Scaling/1(I/p)
  Subtract2/1 -> Gear_ratio/1
  Driveline_viscous_losses/1(O/p) -> Subtract2/2
  Motor/1(O/p) -> Subtract2/1, Scope3/1
  [Vel] -> Abs/1
  PI Controller/1 -> Scope24/1, Motor/2(I/p1), Brake_system/1(I/p)
  [Inputs] -> Subtract/1, Scope18/1, To Workspace/1  "Desired"
  Subtract/1 -> Scope19/1, PI Controller/1  "Error"

== system Motion_planner_Street_Drone/Trajectory Tracker/KM- StreetDrone/Street_Drone/Results1 ==
  Actual brake torque : Subsystem
  Ay&Yaw : Subsystem
  Coordinates : Subsystem
  Fx : Subsystem
  Fy : Subsystem
  Fz : Subsystem
  Steering_angle : Subsystem
  Subsystem1 : Subsystem
  Velocity&Ax : Subsystem
